simulink library "INT_OilPLmp_DD"  (R2016b)
settings: Solver=VariableStepAuto  StartTime=0.0  StopTime=10.0  RelTol=1e-3
settings Model: Creator=xinchangran  LastModifiedBy=xinchangran

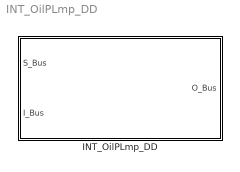
== system INT_OilPLmp_DD ==
  INT_OilPLmp_DD : Subsystem

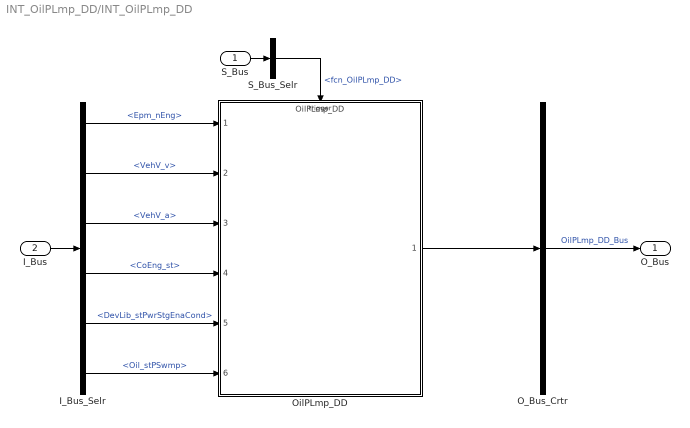
== system INT_OilPLmp_DD/INT_OilPLmp_DD ==
  S_Bus : Inport
  I_Bus : Inport  Port=2
  I_Bus_Selr : BusSelector  OutputSignals=Epm_nEng,VehV_v,VehV_a,CoEng_st,DevLib_stPwrStgEnaCond,Oil_stPSwmp
  O_Bus_Crtr : BusCreator  Inputs=1
  OilPLmp_DD : ModelReference  ModelNameDialog=OilPLmp_DD  SimulationMode=Normal  ModelReferenceVersion=1.212  TriggerPortName=function  TriggerPortTriggerType=function-call  TriggerPortStatesWhenEnabling=held
  S_Bus_Selr : BusSelector  OutputSignals=fcn_OilPLmp_DD
  O_Bus : Outport
  wires:
  S_Bus_Selr/1 -> OilPLmp_DD/Trigger  "<fcn_OilPLmp_DD>"
  S_Bus/1 -> S_Bus_Selr/1
  I_Bus/1 -> I_Bus_Selr/1
  I_Bus_Selr/1 -> OilPLmp_DD/1  "<Epm_nEng>"
  I_Bus_Selr/2 -> OilPLmp_DD/2  "<VehV_v>"
  I_Bus_Selr/3 -> OilPLmp_DD/3  "<VehV_a>"
  I_Bus_Selr/4 -> OilPLmp_DD/4  "<CoEng_st>"
  I_Bus_Selr/5 -> OilPLmp_DD/5  "<DevLib_stPwrStgEnaCond>"
  I_Bus_Selr/6 -> OilPLmp_DD/6  "<Oil_stPSwmp>"
  O_Bus_Crtr/1 -> O_Bus/1  "OilPLmp_DD_Bus"
  OilPLmp_DD/1 -> O_Bus_Crtr/1
